simulink model "radar_lidar_road_double"  (R2021b)
settings: Solver=FixedStepDiscrete  StartTime=0.0  StopTime=10.0  RelTol=1e-3
model workspace (MAT data in the model file):
  firstWarning = 1
  originalScenarioChecksum = '4A544F35B5F16CEB30B2C31E0C92B54A'
libraries: drivingscenarioandsensors x4
(part 1 of 34)
settings Model: Creator=ghisl  LastModifiedBy=ghisl

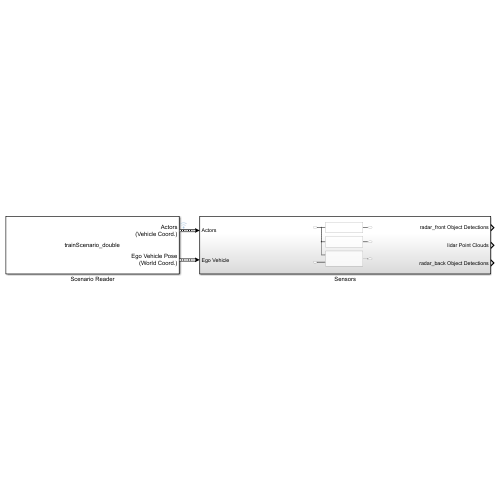
[thumbnail: Simulink's stored preview of the top-level diagram]
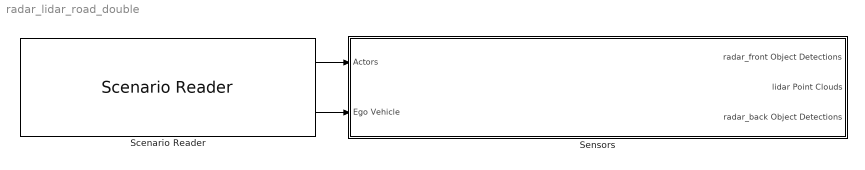
== system radar_lidar_road_double ==
  Scenario Reader : drivingscenarioandsensors/Scenario Reader  ScenarioSource=From file  ScenarioFileName=G:\My Drive\UniBG\CORSI\Laurea Magistrale\2021_2022 - Magistrale Secondo Anno\secondo_semestre\Tirocinio Formativo\tirocinio_PRSE\matlab_stuff\simulink_simulations\trainScenario_double.mat  ScenarioVariableName=scenario  OutputCoordinateSystem=Vehicle coordinates  EgoVehicleSource=Scenario  EgoVehicleActorID=1  OrientVehiclesOnRoad=off  OutputEgoVehiclePose=on  OutputEgoVehicleState=off  SampleTime=0.1  LaneBoundaryOutput=None  LaneBoundaryDistance=0:0.5:9.5  LaneBoundaryLocation=Center of lane markings  BusNameSource=Auto  BusName=BusActors  BusNumActorsSource=Scenario  BusNumActors=100  BusName2Source=Auto  BusName2=BusLaneBoundaries  BusNumLaneBoundariesSource=Scenario  BusNumLaneBoundaries=10  BusName3Source=Auto  BusName3=BusEgoActor  BusName4Source=Auto  BusName4=BusEgoState  ShowCoordinateLabels=on  SimulateUsing=Interpreted execution
  Sensors : Subsystem
  wires:
  Scenario Reader/1 -> Sensors/1(Actors)
  Scenario Reader/2 -> Sensors/2(Ego Vehicle)
